simulink library "BMSI_lib"  (Simulink 7.5)
settings: Solver=ode45  StartTime=0.0  StopTime=10.0  RelTol=1e-3
values from neighbouring files (symbols this model uses):
  pBMSI_bool_HandShakeOverFlag_C = Simulink.Parameter    [BMSI_par.m]
  pBMSI_bool_InterLockOverFlag_C = Simulink.Parameter    [BMSI_par.m]
  pBMSI_bool_StnCfgStOverFlag_C = Simulink.Parameter    [BMSI_par.m]
  pBMSI_mV_DSPInterLowrRngThd_C = Simulink.Parameter    [BMSI_par.m]
  pBMSI_mV_DSPInterUpprRngThd_C = Simulink.Parameter    [BMSI_par.m]
  pBMSI_mV_InterlockDiffThd_C = Simulink.Parameter    [BMSI_par.m]
  pBMSI_mV_InterlockLowrRngThd_C = Simulink.Parameter    [BMSI_par.m]
  pBMSI_mV_InterlockUpprRngThd_C = Simulink.Parameter    [BMSI_par.m]
  pBMSI_pct_LoSOCThd_C = Simulink.Parameter    [BMSI_par.m]
  pBMSI_st_DCChrgrErrSt_C = Simulink.Parameter    [BMSI_par.m]
undefined symbols (not defined in the file or in its folder): ChrgHandShakeTyp, ChrgStationParCnfTyp, FAWBatInsMeasStsTyp, FAWBmsChrgStsTyp, FAWBmsContErrTyp, FAWBMSStsTyp, p_bool_dSPaceEnbl_C, p_bool_False_M, p_bool_True_M
libraries: BaseOperationLib_Browser x116, PES_CZ_FAW x15, simulink x1
(part 2 of 2)

== system BMSI_lib/BMSI/Algo/valid_check14 ==
  Signal : Inport
  Valid : Inport  Port=2
  Switch : BaseOperationLib_Browser/Signal Routing Changed/Switch  Criteria=u2 ~= 0  Threshold=1  InputSameDT=on  OutMin=[]  OutMax=[]  OutDataType=fixdt(1,16,0)  OutScaling=[]  SaturateOnIntegerOverflow=on
  Unit Delay : BaseOperationLib_Browser/Discrete Unchanged /Unit Delay  X0=init  SampleTime=-1
  SignalOut : Outport
  wires:
  Valid/1 -> Switch/2
  Signal/1 -> Switch/1
  Unit Delay/1 -> Switch/3
  Switch/1 -> SignalOut/1, Unit Delay/1

== system BMSI_lib/BMSI/Algo/valid_check2 ==
  Signal : Inport
  Valid : Inport  Port=2
  Switch : BaseOperationLib_Browser/Signal Routing Changed/Switch  Criteria=u2 ~= 0  Threshold=1  InputSameDT=on  OutMin=[]  OutMax=[]  OutDataType=fixdt(1,16,0)  OutScaling=[]  SaturateOnIntegerOverflow=on
  Unit Delay : BaseOperationLib_Browser/Discrete Unchanged /Unit Delay  X0=init  SampleTime=-1
  SignalOut : Outport
  wires:
  Switch/1 -> Unit Delay/1, SignalOut/1
  Unit Delay/1 -> Switch/3
  Signal/1 -> Switch/1
  Valid/1 -> Switch/2

== system BMSI_lib/BMSI/Algo/valid_check3 ==
  Signal : Inport
  Valid : Inport  Port=2
  Switch : BaseOperationLib_Browser/Signal Routing Changed/Switch  Criteria=u2 ~= 0  Threshold=1  InputSameDT=on  OutMin=[]  OutMax=[]  OutDataType=fixdt(1,16,0)  OutScaling=[]  SaturateOnIntegerOverflow=on
  Unit Delay : BaseOperationLib_Browser/Discrete Unchanged /Unit Delay  X0=init  SampleTime=-1
  SignalOut : Outport
  wires:
  Valid/1 -> Switch/2
  Signal/1 -> Switch/1
  Unit Delay/1 -> Switch/3
  Switch/1 -> SignalOut/1, Unit Delay/1

== system BMSI_lib/BMSI/Algo/valid_check4 ==
  Signal : Inport
  Valid : Inport  Port=2
  Switch : BaseOperationLib_Browser/Signal Routing Changed/Switch  Criteria=u2 ~= 0  Threshold=1  InputSameDT=on  OutMin=[]  OutMax=[]  OutDataType=fixdt(1,16,0)  OutScaling=[]  SaturateOnIntegerOverflow=on
  Unit Delay : BaseOperationLib_Browser/Discrete Unchanged /Unit Delay  X0=init  SampleTime=-1
  SignalOut : Outport
  wires:
  Valid/1 -> Switch/2
  Signal/1 -> Switch/1
  Unit Delay/1 -> Switch/3
  Switch/1 -> SignalOut/1, Unit Delay/1

== system BMSI_lib/BMSI/Algo/valid_check5 ==
  Signal : Inport
  Valid : Inport  Port=2
  Switch : BaseOperationLib_Browser/Signal Routing Changed/Switch  Criteria=u2 ~= 0  Threshold=1  InputSameDT=on  OutMin=[]  OutMax=[]  OutDataType=fixdt(1,16,0)  OutScaling=[]  SaturateOnIntegerOverflow=on
  Unit Delay : BaseOperationLib_Browser/Discrete Unchanged /Unit Delay  X0=init  SampleTime=-1
  SignalOut : Outport
  wires:
  Valid/1 -> Switch/2
  Signal/1 -> Switch/1
  Unit Delay/1 -> Switch/3
  Switch/1 -> SignalOut/1, Unit Delay/1

== system BMSI_lib/BMSI/Algo/valid_check6 ==
  Signal : Inport
  Valid : Inport  Port=2
  Switch : BaseOperationLib_Browser/Signal Routing Changed/Switch  Criteria=u2 ~= 0  Threshold=1  InputSameDT=on  OutMin=[]  OutMax=[]  OutDataType=fixdt(1,16,0)  OutScaling=[]  SaturateOnIntegerOverflow=on
  Unit Delay : BaseOperationLib_Browser/Discrete Unchanged /Unit Delay  X0=init  SampleTime=-1
  SignalOut : Outport
  wires:
  Valid/1 -> Switch/2
  Signal/1 -> Switch/1
  Unit Delay/1 -> Switch/3
  Switch/1 -> SignalOut/1, Unit Delay/1

== system BMSI_lib/BMSI/Algo/valid_check7 ==
  Signal : Inport
  Valid : Inport  Port=2
  Switch : BaseOperationLib_Browser/Signal Routing Changed/Switch  Criteria=u2 ~= 0  Threshold=1  InputSameDT=on  OutMin=[]  OutMax=[]  OutDataType=fixdt(1,16,0)  OutScaling=[]  SaturateOnIntegerOverflow=on
  Unit Delay : BaseOperationLib_Browser/Discrete Unchanged /Unit Delay  X0=init  SampleTime=-1
  SignalOut : Outport
  wires:
  Valid/1 -> Switch/2
  Signal/1 -> Switch/1
  Unit Delay/1 -> Switch/3
  Switch/1 -> SignalOut/1, Unit Delay/1

== system BMSI_lib/BMSI/Algo/valid_check8 ==
  Signal : Inport
  Valid : Inport  Port=2
  Switch : BaseOperationLib_Browser/Signal Routing Changed/Switch  Criteria=u2 ~= 0  Threshold=1  InputSameDT=on  OutMin=[]  OutMax=[]  OutDataType=fixdt(1,16,0)  OutScaling=[]  SaturateOnIntegerOverflow=on
  Unit Delay : BaseOperationLib_Browser/Discrete Unchanged /Unit Delay  X0=init  SampleTime=-1
  SignalOut : Outport
  wires:
  Valid/1 -> Switch/2
  Signal/1 -> Switch/1
  Unit Delay/1 -> Switch/3
  Switch/1 -> SignalOut/1, Unit Delay/1

== system BMSI_lib/BMSI/Algo/valid_check9 ==
  Signal : Inport
  Valid : Inport  Port=2
  Switch : BaseOperationLib_Browser/Signal Routing Changed/Switch  Criteria=u2 ~= 0  Threshold=1  InputSameDT=on  OutMin=[]  OutMax=[]  OutDataType=fixdt(1,16,0)  OutScaling=[]  SaturateOnIntegerOverflow=on
  Unit Delay : BaseOperationLib_Browser/Discrete Unchanged /Unit Delay  X0=init  SampleTime=-1
  SignalOut : Outport
  wires:
  Valid/1 -> Switch/2
  Signal/1 -> Switch/1
  Unit Delay/1 -> Switch/3
  Switch/1 -> SignalOut/1, Unit Delay/1

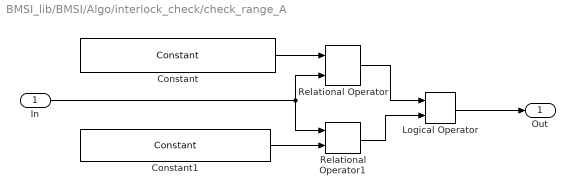
== system BMSI_lib/BMSI/Algo/interlock_check/check_range_A ==
  In : Inport
  Constant : BaseOperationLib_Browser/Sources&Sinks/Constant  Value=pBMSI_mV_InterlockUpprRngThd_C  OutMin=[]  OutMax=[]  OutDataType=fixdt(1, 16)  ConRadixGroup=Use specified scaling  OutScaling=2^0  OutDataTypeStr=Inherit: Inherit from 'Constant value'
  Constant1 : BaseOperationLib_Browser/Sources&Sinks/Constant  Value=pBMSI_mV_InterlockLowrRngThd_C  OutMin=[]  OutMax=[]  OutDataType=fixdt(1, 16)  ConRadixGroup=Use specified scaling  OutScaling=2^0  OutDataTypeStr=Inherit: Inherit from 'Constant value'
  Logical Operator : BaseOperationLib_Browser/Logic Operations Changed/Logical Operator  Operator=AND  Inputs=2  AllPortsSameDT=on  OutDataTypeMode=Specify via dialog  LogicDataType=PDT_Bool  OutDataTypeStr=PDT_Bool
  Relational Operator : BaseOperationLib_Browser/Logic Operations Changed/Relational Operator  Operator=>=  InputSameDT=on  LogicOutDataTypeMode=Specify via dialog  LogicDataType=PDT_Bool  OutDataTypeStr=PDT_Bool
  Relational Operator1 : BaseOperationLib_Browser/Logic Operations Changed/Relational Operator  Operator=>=  InputSameDT=on  LogicOutDataTypeMode=Specify via dialog  LogicDataType=PDT_Bool  OutDataTypeStr=PDT_Bool
  Out : Outport
  wires:
  Constant/1 -> Relational Operator/1
  Constant1/1 -> Relational Operator1/2
  Relational Operator/1 -> Logical Operator/1
  Relational Operator1/1 -> Logical Operator/2
  Logical Operator/1 -> Out/1
  In/1 -> Relational Operator/2, Relational Operator1/1

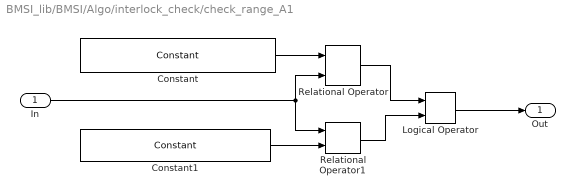
== system BMSI_lib/BMSI/Algo/interlock_check/check_range_A1 ==
  In : Inport
  Constant : BaseOperationLib_Browser/Sources&Sinks/Constant  Value=pBMSI_mV_DSPInterUpprRngThd_C  OutMin=[]  OutMax=[]  OutDataType=fixdt(1, 16)  ConRadixGroup=Use specified scaling  OutScaling=2^0  OutDataTypeStr=Inherit: Inherit from 'Constant value'
  Constant1 : BaseOperationLib_Browser/Sources&Sinks/Constant  Value=pBMSI_mV_DSPInterLowrRngThd_C  OutMin=[]  OutMax=[]  OutDataType=fixdt(1, 16)  ConRadixGroup=Use specified scaling  OutScaling=2^0  OutDataTypeStr=Inherit: Inherit from 'Constant value'
  Logical Operator : BaseOperationLib_Browser/Logic Operations Changed/Logical Operator  Operator=AND  Inputs=2  AllPortsSameDT=on  OutDataTypeMode=Specify via dialog  LogicDataType=PDT_Bool  OutDataTypeStr=PDT_Bool
  Relational Operator : BaseOperationLib_Browser/Logic Operations Changed/Relational Operator  Operator=>=  InputSameDT=on  LogicOutDataTypeMode=Specify via dialog  LogicDataType=PDT_Bool  OutDataTypeStr=PDT_Bool
  Relational Operator1 : BaseOperationLib_Browser/Logic Operations Changed/Relational Operator  Operator=>=  InputSameDT=on  LogicOutDataTypeMode=Specify via dialog  LogicDataType=PDT_Bool  OutDataTypeStr=PDT_Bool
  Out : Outport
  wires:
  In/1 -> Relational Operator1/1, Relational Operator/2
  Logical Operator/1 -> Out/1
  Relational Operator1/1 -> Logical Operator/2
  Relational Operator/1 -> Logical Operator/1
  Constant1/1 -> Relational Operator1/2
  Constant/1 -> Relational Operator/1

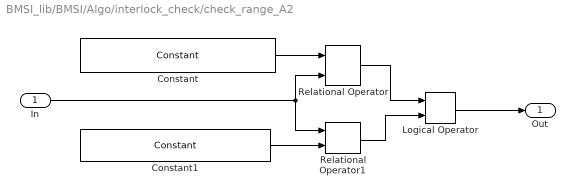
== system BMSI_lib/BMSI/Algo/interlock_check/check_range_A2 ==
  In : Inport
  Constant : BaseOperationLib_Browser/Sources&Sinks/Constant  Value=pBMSI_mV_DSPInterUpprRngThd_C  OutMin=[]  OutMax=[]  OutDataType=fixdt(1, 16)  ConRadixGroup=Use specified scaling  OutScaling=2^0  OutDataTypeStr=Inherit: Inherit from 'Constant value'
  Constant1 : BaseOperationLib_Browser/Sources&Sinks/Constant  Value=pBMSI_mV_DSPInterLowrRngThd_C  OutMin=[]  OutMax=[]  OutDataType=fixdt(1, 16)  ConRadixGroup=Use specified scaling  OutScaling=2^0  OutDataTypeStr=Inherit: Inherit from 'Constant value'
  Logical Operator : BaseOperationLib_Browser/Logic Operations Changed/Logical Operator  Operator=AND  Inputs=2  AllPortsSameDT=on  OutDataTypeMode=Specify via dialog  LogicDataType=PDT_Bool  OutDataTypeStr=PDT_Bool
  Relational Operator : BaseOperationLib_Browser/Logic Operations Changed/Relational Operator  Operator=>=  InputSameDT=on  LogicOutDataTypeMode=Specify via dialog  LogicDataType=PDT_Bool  OutDataTypeStr=PDT_Bool
  Relational Operator1 : BaseOperationLib_Browser/Logic Operations Changed/Relational Operator  Operator=>=  InputSameDT=on  LogicOutDataTypeMode=Specify via dialog  LogicDataType=PDT_Bool  OutDataTypeStr=PDT_Bool
  Out : Outport
  wires:
  Constant/1 -> Relational Operator/1
  Constant1/1 -> Relational Operator1/2
  Relational Operator/1 -> Logical Operator/1
  Relational Operator1/1 -> Logical Operator/2
  Logical Operator/1 -> Out/1
  In/1 -> Relational Operator/2, Relational Operator1/1

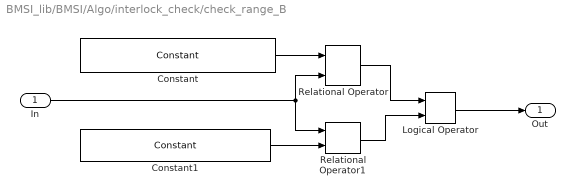
== system BMSI_lib/BMSI/Algo/interlock_check/check_range_B ==
  In : Inport
  Constant : BaseOperationLib_Browser/Sources&Sinks/Constant  Value=pBMSI_mV_InterlockUpprRngThd_C  OutMin=[]  OutMax=[]  OutDataType=fixdt(1, 16)  ConRadixGroup=Use specified scaling  OutScaling=2^0  OutDataTypeStr=Inherit: Inherit from 'Constant value'
  Constant1 : BaseOperationLib_Browser/Sources&Sinks/Constant  Value=pBMSI_mV_InterlockLowrRngThd_C  OutMin=[]  OutMax=[]  OutDataType=fixdt(1, 16)  ConRadixGroup=Use specified scaling  OutScaling=2^0  OutDataTypeStr=Inherit: Inherit from 'Constant value'
  Logical Operator : BaseOperationLib_Browser/Logic Operations Changed/Logical Operator  Operator=AND  Inputs=2  AllPortsSameDT=on  OutDataTypeMode=Specify via dialog  LogicDataType=PDT_Bool  OutDataTypeStr=PDT_Bool
  Relational Operator : BaseOperationLib_Browser/Logic Operations Changed/Relational Operator  Operator=>=  InputSameDT=on  LogicOutDataTypeMode=Specify via dialog  LogicDataType=PDT_Bool  OutDataTypeStr=PDT_Bool
  Relational Operator1 : BaseOperationLib_Browser/Logic Operations Changed/Relational Operator  Operator=>=  InputSameDT=on  LogicOutDataTypeMode=Specify via dialog  LogicDataType=PDT_Bool  OutDataTypeStr=PDT_Bool
  Out : Outport
  wires:
  Constant/1 -> Relational Operator/1
  Constant1/1 -> Relational Operator1/2
  Relational Operator/1 -> Logical Operator/1
  Relational Operator1/1 -> Logical Operator/2
  Logical Operator/1 -> Out/1
  In/1 -> Relational Operator/2, Relational Operator1/1
